simulink model "ac"  (R2018a)
settings: Solver=FixedStepAuto  StartTime=0.0  StopTime=3  FixedStep=0.01  RelTol=1e-3
undefined symbols (not defined in the file or in its folder): sigbuilder_block
libraries: aerolibactuator x5, simulink x2
settings Model: Creator=mengc  LastModifiedBy=mengc

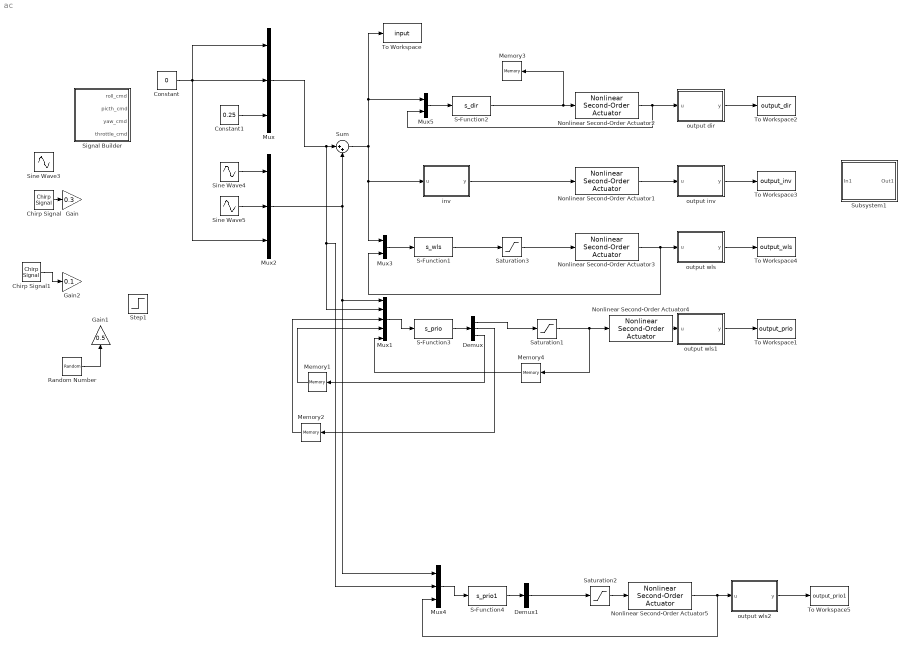
== system ac ==
  Chirp Signal : simulink/Sources/Chirp Signal  f1=1  T=3  f2=5
  Chirp Signal1 : simulink/Sources/Chirp Signal  f1=1  T=3  f2=10
  Constant : Constant  Value=0  SampleTime=0.01
  Constant1 : Constant  Value=0.25  SampleTime=0.01
  Demux : Demux  Outputs=3
  Demux1 : Demux  Outputs=1
  Gain : Gain  Gain=0.3
  Gain1 : Gain  Gain=0.5
  Gain2 : Gain  Gain=0.1
  Memory1 : Memory  InitialCondition=[0;0;0]  InheritSampleTime=on  LinearizeAsDelay=on
  Memory2 : Memory  InitialCondition=[0;0;0]  InheritSampleTime=on  LinearizeAsDelay=on
  Memory3 : Memory  InitialCondition=[0;0;0;0]  InheritSampleTime=on  LinearizeAsDelay=on
  Memory4 : Memory  InitialCondition=[0;0;0;0]  InheritSampleTime=on  LinearizeAsDelay=on
  Mux : Mux  Inputs=3
  Mux1 : Mux  Inputs=5
  Mux2 : Mux  Inputs=3
  Mux3 : Mux  Inputs=2
  Mux4 : Mux  Inputs=3
  Mux5 : Mux  Inputs=2
  Nonlinear Second-Order Actuator{1..5} (5 alike) : aerolibactuator/Nonlinear Second-Order Actuator  wn_fin=200  z_fin=0.7  fin_max=20*pi/180  fin_min=-20*pi/180  fin_maxrate=500*pi/180  fin_act_0=0  fin_act_vel=0
      settings: SourceProductName=Aerospace Blockset  SourceProductBaseCode=AE
  Random Number : RandomNumber  Variance=0.1  SampleTime=0.01
  S-Function1 : S-Function  FunctionName=s_wls  SFunctionDeploymentMode=off  EnableBusSupport=off
  S-Function2 : S-Function  FunctionName=s_dir  SFunctionDeploymentMode=off  EnableBusSupport=off
  S-Function3 : S-Function  FunctionName=s_prio  SFunctionDeploymentMode=off  EnableBusSupport=off
  S-Function4 : S-Function  FunctionName=s_prio1  SFunctionDeploymentMode=off  EnableBusSupport=off
  Saturation1 : Saturate  UpperLimit=[1;1;1;1]*20*pi/180  LowerLimit=-[1;1;1;1]*20*pi/180
  Saturation2 : Saturate  UpperLimit=[1;1;1;1]*20*pi/180  LowerLimit=-[1;1;1;1]*20*pi/180
  Saturation3 : Saturate  UpperLimit=[1;1;1;1]*20*pi/180  LowerLimit=-[1;1;1;1]*20*pi/180
  Signal Builder : Subsystem  Tag=STV Subsys  LoadFcn=sigbuilder_block('load');  StartFcn=sigbuilder_block('start');  StopFcn=sigbuilder_block('stop');  ClipboardFcn=sigbuilder_block('clipboard');  mask(Sigbuilder block){tuvar=[0:10]}
      mask help: Simulink:masks:SigbuilderBlock_MD
      mask init:
      | if ~strcmp(get_param(bdroot(gcbh),'SimulationStatus'),'stopped') tuvar = sigbuilder_block('maskInit'); end
      settings: CopyFcn=sigbuilder_block('copy');  DeleteFcn=sigbuilder_block('delete');  ModelCloseFcn=sigbuilder_block('modelClose');  PreSaveFcn=sigbuilder_block('preSave');  PauseFcn=sigbuilder_block('pause');  ContinueFcn=sigbuilder_block('continue');  NameChangeFcn=sigbuilder_block('namechange');  OpenFcn=sigbuilder_block('open',[42.75 46.5 943.5 423.75 ]);  CloseFcn=sigbuilder_block('close');
      mask Display: plot(0, 0, 100, 100,[2, 2, 32, 32, 2], [68, 8, 8, 68, 68],[32, 2], [38, 38], [32, 19, 2],[53, 60, 44], [32, 17, 17, 2],[16, 16, 31, 31]);txt = getActiveGroup(gcbh);text(2, 100, txt,'verticalAlignment', 'top');
  Sine Wave3 : Sin  Amplitude=0.34  Frequency=2*pi/2  SampleTime=0.01
  Sine Wave4 : Sin  Amplitude=0.34  Frequency=2*pi/2  Phase=pi/2  SampleTime=0
  Sine Wave5 : Sin  Amplitude=0.34  Frequency=2*pi/2  SampleTime=0.01
  Step1 : Step  After=0.4  SampleTime=0
  Subsystem1 : Subsystem
  Sum : Sum  Inputs=|++
  To Workspace : ToWorkspace  VariableName=input  SaveFormat=Timeseries  SampleTime=-1
  To Workspace1 : ToWorkspace  VariableName=output_prio  SaveFormat=Timeseries  SampleTime=-1
  To Workspace2 : ToWorkspace  VariableName=output_dir  SaveFormat=Timeseries  SampleTime=-1
  To Workspace3 : ToWorkspace  VariableName=output_inv  SaveFormat=Timeseries  SampleTime=-1
  To Workspace4 : ToWorkspace  VariableName=output_wls  SaveFormat=Timeseries  SampleTime=-1
  To Workspace5 : ToWorkspace  VariableName=output_prio1  SaveFormat=Timeseries  SampleTime=-1
  inv : MATLAB Function  TreatAsAtomicUnit=on
  output dir : MATLAB Function  TreatAsAtomicUnit=on  SystemSampleTime=0.01
  output inv : MATLAB Function  TreatAsAtomicUnit=on  SystemSampleTime=0.01
  output wls : MATLAB Function  TreatAsAtomicUnit=on  SystemSampleTime=0.01
  output wls1 : MATLAB Function  TreatAsAtomicUnit=on  SystemSampleTime=0.01
  output wls2 : MATLAB Function  TreatAsAtomicUnit=on  SystemSampleTime=0.01
  wires:
  S-Function1/1 -> Saturation3/1
  output inv/1(y) -> To Workspace3/1
  Mux3/1 -> S-Function1/1
  S-Function2/1 -> Memory3/1, Nonlinear Second-Order Actuator2/1
  output wls/1(y) -> To Workspace4/1
  Mux/1 -> Mux4/2, Mux1/2, Sum/1
  inv/1(y) -> Nonlinear Second-Order Actuator1/1
  output dir/1(y) -> To Workspace2/1
  Mux5/1 -> S-Function2/1
  Chirp Signal/1 -> Gain/1
  Random Number/1 -> Gain1/1
  Nonlinear Second-Order Actuator1/1 -> output inv/1(u)
  Nonlinear Second-Order Actuator2/1 -> Mux5/2, output dir/1(u)
  Chirp Signal1/1 -> Gain2/1
  Constant/1 -> Mux/2, Mux2/3, Mux/1
  Mux1/1 -> S-Function3/1
  output wls1/1(y) -> To Workspace1/1
  S-Function3/1 -> Demux/1
  Sum/1 -> Mux5/1, To Workspace/1, Mux3/1, inv/1(u)
  Nonlinear Second-Order Actuator3/1 -> Mux3/2, output wls/1(u)
  Nonlinear Second-Order Actuator4/1 -> output wls1/1(u)
  Saturation3/1 -> Nonlinear Second-Order Actuator3/1
  Sine Wave4/1 -> Mux2/1
  Sine Wave5/1 -> Mux2/2
  Constant1/1 -> Mux/3
  Demux/3 -> Memory1/1
  Demux/2 -> Memory2/1
  Memory2/1 -> Mux1/3
  Memory1/1 -> Mux1/4
  Demux/1 -> Saturation1/1
  S-Function4/1 -> Demux1/1
  Mux2/1 -> Mux1/1, Mux4/1, Sum/2
  output wls2/1(y) -> To Workspace5/1
  Nonlinear Second-Order Actuator5/1 -> Mux4/3, output wls2/1(u)
  Mux4/1 -> S-Function4/1
  Saturation2/1 -> Nonlinear Second-Order Actuator5/1
  Demux1/1 -> Saturation2/1
  Saturation1/1 -> Memory4/1, Nonlinear Second-Order Actuator4/1
  Memory4/1 -> Mux1/5

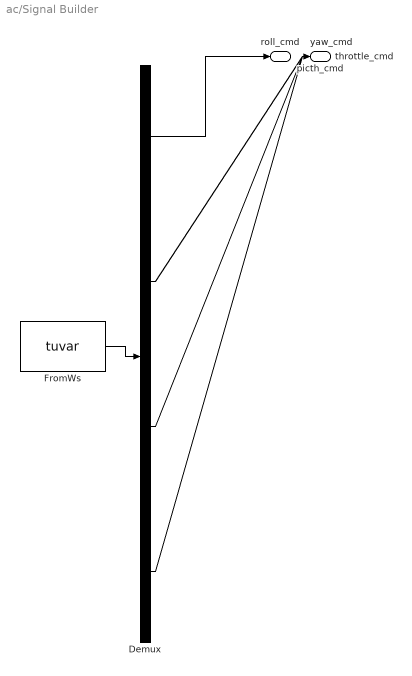
== system ac/Signal Builder ==
  Demux : Demux  Tag=STV Demux
  FromWs : FromWorkspace  Tag=STV FromWs  VariableName=tuvar  SampleTime=0
      SigBuilderData=|
      | common.afterFinalStr = 'Extrapolate'
      | common.sampleTime = 0
      | dataSet.timeRange = [0 100]
      | dataSet.name = 'Group 1'
      | sbobj.Groups.Name = 'Group 1'
      | sbobj.Groups.Signals(1).Name = 'roll_cmd'
      | sbobj.Groups.Signals(1).XData = [0 5 100]
      | sbobj.Groups.Signals(1).YData = [0 0.25 0.25]
      | sbobj.Groups.Signals(2).Name = 'picth_cmd'
      | sbobj.Groups.Signals(2).XData = [0 30 30 100]
      | sbobj.Groups.Signals(2).YData = [-0.0045 -0.0045 0.3 0.3]
      | sbobj.Groups.Signals(3).Name = 'yaw_cmd'
      | sbobj.Groups.Signals(3).XData = [0 30 30 100]
      | sbobj.Groups.Signals(3).YData = [0.0779 0.0779 0.2 0.2]
      | sbobj.Groups.Signals(4).Name = 'throttle_cmd'
      | sbobj.Groups.Signals(4).XData = [0 100]
      | sbobj.Groups.Signals(4).YData = [0 0]
      | sbobj.Groups.TimeRange = [0 100]
  roll_cmd : Outport  Tag=STV Outport
  picth_cmd : Outport  Tag=STV Outport  Port=2
  yaw_cmd : Outport  Tag=STV Outport  Port=3
  throttle_cmd : Outport  Tag=STV Outport  Port=4
  wires:
  Demux/1 -> roll_cmd/1
  FromWs/1 -> Demux/1
  Demux/2 -> picth_cmd/1
  Demux/3 -> yaw_cmd/1
  Demux/4 -> throttle_cmd/1

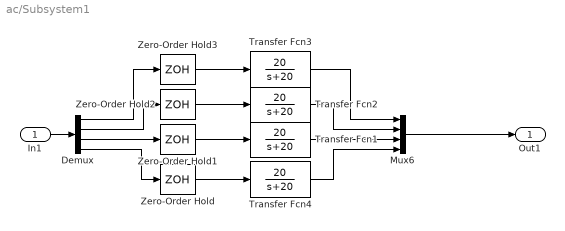
== system ac/Subsystem1 ==
  In1 : Inport
  Demux : Demux
  Mux6 : Mux
  Transfer Fcn{1..4} (4 alike) : TransferFcn  Numerator=[20]  Denominator=[1 20]
  Zero-Order Hold{,1..3} (4 alike) : ZeroOrderHold  SampleTime=-1
  Out1 : Outport
  wires:
  Demux/3 -> Zero-Order Hold1/1
  Zero-Order Hold2/1 -> Transfer Fcn2/1
  Transfer Fcn2/1 -> Mux6/2
  Demux/1 -> Zero-Order Hold3/1
  Transfer Fcn3/1 -> Mux6/1
  Transfer Fcn4/1 -> Mux6/4
  Zero-Order Hold/1 -> Transfer Fcn4/1
  Transfer Fcn1/1 -> Mux6/3
  Zero-Order Hold1/1 -> Transfer Fcn1/1
  Demux/4 -> Zero-Order Hold/1
  Zero-Order Hold3/1 -> Transfer Fcn3/1
  Demux/2 -> Zero-Order Hold2/1
  In1/1 -> Demux/1
  Mux6/1 -> Out1/1

== matlab function ac/output wls1 ==
  data: u input; y output
function y = fcn(u)
% u(1)=Constrain(u(1),-0.3491,0.3491);
% u(2)=Constrain(u(2),-0.3491,0.3491);
% u(3)=Constrain(u(3),-0.3491,0.3491);
% u(4)=Constrain(u(4),-0.3491,0.3491);
B=[-0.5   0       0.5   0;
    0  -0.5    0       0.5;
    0.25   0.25   0.25   0.25];
B=[-0.5393   0       0.5393   0;
     0  -0.5393    0       0.5393;
    0.2099   0.2099   0.2099   0.2099];
y = B*[u(1);u(2);u(3);u(4)];

== matlab function ac/output wls2 ==
  data: u input; y output
function y = fcn(u)
% u(1)=Constrain(u(1),-0.3491,0.3491);
% u(2)=Constrain(u(2),-0.3491,0.3491);
% u(3)=Constrain(u(3),-0.3491,0.3491);
% u(4)=Constrain(u(4),-0.3491,0.3491);
B=[-0.5   0       0.5   0;
    0  -0.5    0       0.5;
    0.25   0.25   0.25   0.25];
B=[-0.5393   0       0.5393   0;
     0  -0.5393    0       0.5393;
    0.2099   0.2099   0.2099   0.2099];
y = B*[u(1);u(2);u(3);u(4)];

== matlab function ac/output dir ==
  data: u input; y output
function y = fcn(u)
% u(1)=Constrain(u(1),-0.3491,0.3491);
% u(2)=Constrain(u(2),-0.3491,0.3491);
% u(3)=Constrain(u(3),-0.3491,0.3491);
% u(4)=Constrain(u(4),-0.3491,0.3491);
B=[-0.5   0       0.5   0;
    0  -0.5    0       0.5;
    0.25   0.25   0.25   0.25];
y = B*[u(1);u(2);u(3);u(4)];

== matlab function ac/output inv ==
  data: u input; y output
function y = fcn(u)
% u(1)=Constrain(u(1),-0.3491,0.3491);
% u(2)=Constrain(u(2),-0.3491,0.3491);
% u(3)=Constrain(u(3),-0.3491,0.3491);
% u(4)=Constrain(u(4),-0.3491,0.3491);
B=[-0.5   0       0.5   0;
    0  -0.5    0       0.5;
    0.25   0.25   0.25   0.25];
B=[-0.5393   0       0.5393   0;
     0  -0.5393    0       0.5393;
    0.2099   0.2099   0.2099   0.2099];
y = B*[u(1);u(2);u(3);u(4)];

== matlab function ac/output wls ==
  data: u input; y output
function y = fcn(u)
% u(1)=Constrain(u(1),-0.3491,0.3491);
% u(2)=Constrain(u(2),-0.3491,0.3491);
% u(3)=Constrain(u(3),-0.3491,0.3491);
% u(4)=Constrain(u(4),-0.3491,0.3491);
B=[-0.5   0       0.5   0;
    0  -0.5    0       0.5;
    0.25   0.25   0.25   0.25];
B=[-0.5393   0       0.5393   0;
     0  -0.5393    0       0.5393;
    0.2099   0.2099   0.2099   0.2099];
y = B*[u(1);u(2);u(3);u(4)];

== matlab function ac/inv ==
  data: u input; y output
function y = fcn(u)
U = [u(1);u(2);u(3)];
% M=crossover_point([0;0;0],e);
% if (norm(e)>norm(M))
%     U=M;
% else
%     U=e;
% end 
B=[-0.5   0       0.5   0;
    0  -0.5    0       0.5;
    0.25   0.25   0.25   0.25];
B=[-0.5393   0       0.5393   0;
     0  -0.5393    0       0.5393;
    0.2099   0.2099   0.2099   0.2099];
% B=[-0.5393   0       0.5393   0;
%      0  -0.5393    0       0.5393;
%     0.2099   0.2099   0.2099   0.2099];
% u(1)=Constrain(u(1),umin(1),umax(1));
% u(2)=Constrain(u(2),umin(2),umax(2));
% u(3)=Constrain(u(3),umin(3),umax(3));
% u(4)=Constrain(u(4),umin(4),umax(4));
c=pinv(B)*U;
y=[c(1);c(2);c(3);c(4)];
